simulink model "Task2_Imbissbude"  (R2018b)
settings: Solver=VariableStepAuto  StartTime=0.0  StopTime=10000  RelTol=1e-3
undefined symbols (not defined in the file): m, n
settings Model: Creator=Dano  LastModifiedBy=Dano

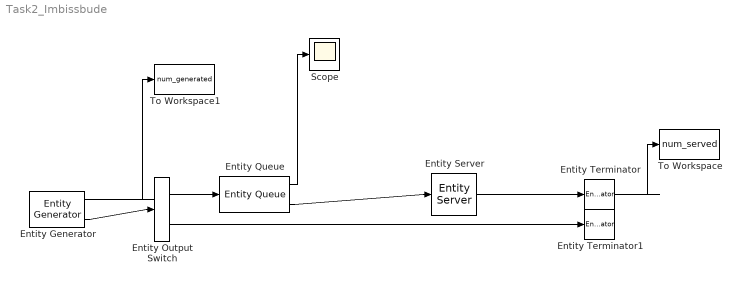
== system Task2_Imbissbude ==
  Entity Output Switch : EntityOutputSwitch  InputPortMessageModes=m  OutputPortMessageModes=m,m  SwitchAttributeName=Attribute1
  Entity Generator : EntityGenerator  OutputPortMessageModes=n,m  TimeSource=MATLAB action  IntergenerationTimeAction=|  NumberEntitiesDeparted=on  EntityType=Structured  EntityTypeName=Entity
      | persistent z
      | if isempty(z)
      |     z = 0;
      |     rng(1000);
      | end
      | 
      | lambda = 0.3;
      | dt = exprnd(1/lambda);
      settings: OutputPortMap=o0,o3
  Entity Queue : EntityQueue  InputPortMessageModes=m  OutputPortMessageModes=n,m  Capacity=seats  AverageQueueLength=on
      settings: OutputPortMap=o3,o5
  Entity Server : EntityServer  InputPortMessageModes=m  OutputPortMessageModes=m  Capacity=1  ServiceTimeSource=MATLAB action  ServiceTimeAction=|
      | persistent z
      | if isempty(z)
      |     z = 0;
      |     rng(2000);
      | end
      | 
      | ts = 2;
      | 
      | dt = exprnd(ts);
  Entity Terminator : EntityTerminator  InputPortMessageModes=m  NumberEntitiesArrived=on
      settings: OutputPortMap=o0
  Entity Terminator1 : EntityTerminator  InputPortMessageModes=m
  Scope : Scope
  To Workspace : ToWorkspace  VariableName=num_served  SampleTime=-1
  To Workspace1 : ToWorkspace  VariableName=num_generated  SampleTime=-1
  wires:
  Entity Queue/2 -> Entity Server/1
  Entity Server/1 -> Entity Terminator/1
  Entity Generator/1 -> To Workspace1/1
  Entity Terminator/1 -> To Workspace/1
  Entity Queue/1 -> Scope/1
  Entity Generator/2 -> Entity Output Switch/1
  Entity Output Switch/1 -> Entity Queue/1
  Entity Output Switch/2 -> Entity Terminator1/1
